simulink model "demodulator_metop_r"  (R2024b)
settings: Solver=FixedStepDiscrete  StartTime=0.0  StopTime=Inf  RelTol=1e-3
libraries: dspsigops x2, commsync2 x2, commrfcorlib x1, commfilt2 x1
settings Model: Creator=Lenovo  LastModifiedBy=Lenovo
settings OptimizationCC: SimCompilerOptimization=on

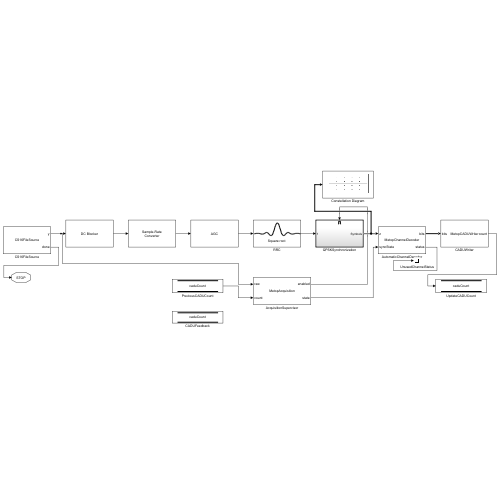
[thumbnail: Simulink's stored preview of the top-level diagram]
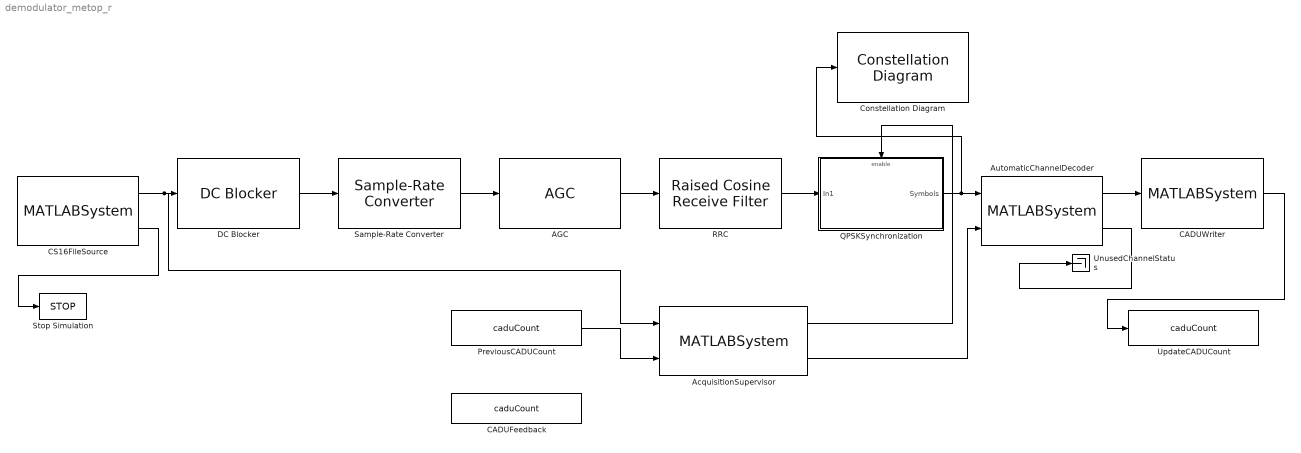
== system demodulator_metop_r ==
  AGC : commrfcorlib/AGC  LegacyMode=off  DetectorMethod=Rectifier  LoopMethod=Linear  UpdatePeriod=100  StepSize=0.1  AdaptationStepSize=0.01  DesiredOutputPower=1  AveragingLength=1024  MaximumGain=30  MaxPowerGain=60  GainOutputPort=off  InputPowerOutputPort=off  SimulateUsing=Code generation
  AcquisitionSupervisor : MATLABSystem  System=MetopAcquisition  FramePeriod=92160 / 10e6  SimulateUsing=Code generation
      mask Type: MetopAcquisition
      mask Display:
      | disp('MetopAcquisition');
      | port_label('input',1,'raw');
      | port_label('input',2,'count');
      | port_label('output',1,'enabled');
      | port_label('output',2,'state');
  AutomaticChannelDecoder : MATLABSystem  System=MetopChannelDecoder  SoftDecision=true  TracebackDepth=96  FramePeriod=92160 / 10e6  SearchInterval=10
      mask Type: MetopChannelDecoder
      mask Display:
      | disp('MetopChannelDecoder');
      | port_label('input',1,'z');
      | port_label('input',2,'syncState');
      | port_label('output',1,'bits');
      | port_label('output',2,'status');
  CADUFeedback : DataStoreMemory  DataStoreName=caduCount  WriteAfterWriteMsg=warning  InitialValue=uint32(0)  ShowAdditionalParam=off  OutDataTypeStr=uint32  Dimensions=1
  CADUWriter : MATLABSystem  System=MetopCADUWriter  Filename=out/metop.cadu
      mask Type: MetopCADUWriter
      mask Display:
      | disp('MetopCADUWriter');
      | port_label('input',1,'bits');
      | port_label('output',1,'count');
  CS16FileSource : MATLABSystem  System=CS16FileSource  Filename=Metop_20260731_1022.cs16  SampleRate=10e6  SamplesPerFrame=92160  Normalize=true  StartTimeSeconds=0
      mask Type: CS16FileSource
      mask Display:
      | disp('CS16FileSource');
      | port_label('output',1,'y');
      | port_label('output',2,'done');
  Constellation Diagram : ConstellationDiagram  WindowPosition=[42.000000,30.000000,600.000000,600.000000,]  Visible=on  ScopeFrameLocation=window  SymbolsToDisplaySource=Property  SymbolsToDisplay=2000  XLimits=[-4.23,4.53]  YLimits=[-4.23,3.84]
  DC Blocker : dspsigops/DC Blocker  Algorithm=IIR  NormalizedBandwidth=0.001  Length=8  Order=6  SimulateUsing=Code generation
      settings: LibrarySourceBlock=commfilt2/DC Blocker
  PreviousCADUCount : DataStoreRead  Priority=1  DataStoreName=caduCount  SampleTime=92160/10e6  IndexOptions=Index vector (dialog)  Indices=1  OutputSizes=1
  QPSKSynchronization : Subsystem  TreatAsAtomicUnit=on
  RRC : commfilt2/Raised Cosine Receive Filter  filtType=Square root  R=0.5  filtSpan=10  N=2  downFactor=1  downOffset=0  filterGain=1  InputProcessing=Columns as channels (frame based)  RateOptions=Enforce single-rate processing  framing=Mute  checkCoeff=off  variableName=rcRxFilt  currentFiltSpan=10  D=5  inputOffset=0  sampMode=Mute  saveAsFlag=0  rateMode=Downsampling  checkGain=Normalized  launchFVT=on  roundingMode=Floor  overflowMode=off  coeffDataTypeStr=Inherit: Same word length as input  coeffMin=[]  coeffMax=[]  coeffLastDataTypeStr=Inherit: Same word length as input  accumDataTypeStr=Inherit: Same as product output  accumLastDataTypeStr=Inherit: Same as product output  outputDataTypeStr=Inherit: Same as accumulator  outputMin=[]  outputMax=[]  outputLastDataTypeStr=Inherit: Same as accumulator
  Sample-Rate Converter : dspsigops/Sample-Rate Converter  InputSampleRate=10e6  OutputSampleRate=14e6/3  OutputRateTolerance=0  Bandwidth=3.8e6  StopbandAttenuation=80  AllowArbitraryInputLength=off  SimulateUsing=Code generation
  Stop Simulation : Stop
  UnusedChannelStatus : Terminator
  UpdateCADUCount : DataStoreWrite  Priority=2  DataStoreName=caduCount  IndexOptions=Index vector (dialog)  Indices=1  OutputSizes=1
  wires:
  PreviousCADUCount/1 -> AcquisitionSupervisor/2
  CS16FileSource/1 -> DC Blocker/1, AcquisitionSupervisor/1
  CADUWriter/1 -> UpdateCADUCount/1
  AcquisitionSupervisor/2 -> AutomaticChannelDecoder/2
  AutomaticChannelDecoder/1 -> CADUWriter/1
  AGC/1 -> RRC/1
  DC Blocker/1 -> Sample-Rate Converter/1
  CS16FileSource/2 -> Stop Simulation/1
  Sample-Rate Converter/1 -> AGC/1
  AutomaticChannelDecoder/2 -> UnusedChannelStatus/1
  AcquisitionSupervisor/1 -> QPSKSynchronization/Enable
  QPSKSynchronization/1(Symbols) -> AutomaticChannelDecoder/1, Constellation Diagram/1
  RRC/1 -> QPSKSynchronization/1(In1)

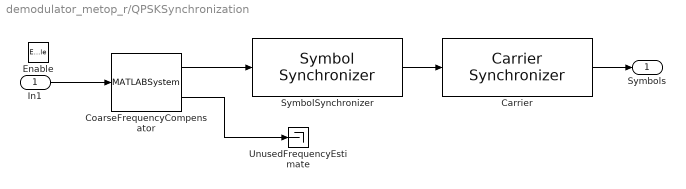
== system demodulator_metop_r/QPSKSynchronization ==
  In1 : Inport
  Enable : EnablePort  StatesWhenEnabling=reset  PropagateVarSize=During execution
  Carrier : commsync2/Carrier Synchronizer  Modulation=QPSK  ModulationPhaseOffset=Auto  CustomPhaseOffset=0  SamplesPerSymbol=1  DampingFactor=0.707  NormalizedLoopBandwidth=0.002  EstimatedPhaseErrorOutputPort=off  SimulateUsing=Code generation
  CoarseFrequencyCompensator : MATLABSystem  System=comm.CoarseFrequencyCompensator  Modulation=QPSK  Algorithm=FFT-based  FrequencyResolution=100  MaximumFrequencyOffset=5e3  SamplesPerSymbol=4  EstimatedFreqOffsetPort=on  SimulateUsing=Code generation
      mask Type: comm.CoarseFrequencyCompensator
      mask Display:
      | disp(['Coarse' char(10) 'Frequency' char(10) 'Compensator']);
      | port_label('output',1,'Out');
      | port_label('output',2,'FreqEst');
  SymbolSynchronizer : commsync2/Symbol Synchronizer  Modulation=PAM/PSK/QAM  TimingErrorDetector=Gardner (non-data-aided)  SamplesPerSymbol=2  DampingFactor=1  NormalizedLoopBandwidth=0.003  DetectorGain=5.4  TimingErrorOutputPort=off  SimulateUsing=Code generation
  UnusedFrequencyEstimate : Terminator
  Symbols : Outport
      settings: VarSizeSig=Yes
  wires:
  Carrier/1 -> Symbols/1
  In1/1 -> CoarseFrequencyCompensator/1
  SymbolSynchronizer/1 -> Carrier/1
  CoarseFrequencyCompensator/2 -> UnusedFrequencyEstimate/1
  CoarseFrequencyCompensator/1 -> SymbolSynchronizer/1
